simulink model "TST_Rail_MonMeUn"  (R2016b)
settings: Solver=FixedStepDiscrete  StartTime=0.0  StopTime=simTime  FixedStep=sampleTime  RelTol=1e-3
values from neighbouring files (symbols this model uses):
  testCase = 1    [initTST_Rail_MonMeUn_001.m]    (also in initTST_Rail_MonMeUn_002.m = 2; initTST_Rail_MonMeUn_003.m = 3; initTST_Rail_MonMeUn_004.m = 4; initTST_Rail_MonMeUn_005.m = 5)
libraries: simulink x91, UnitTest_Lib x81
(part 1 of 5)
settings Model: Creator=zhengjinyan  LastModifiedBy=zhengjinyan
settings DebuggingCC: SignalRangeChecking=error

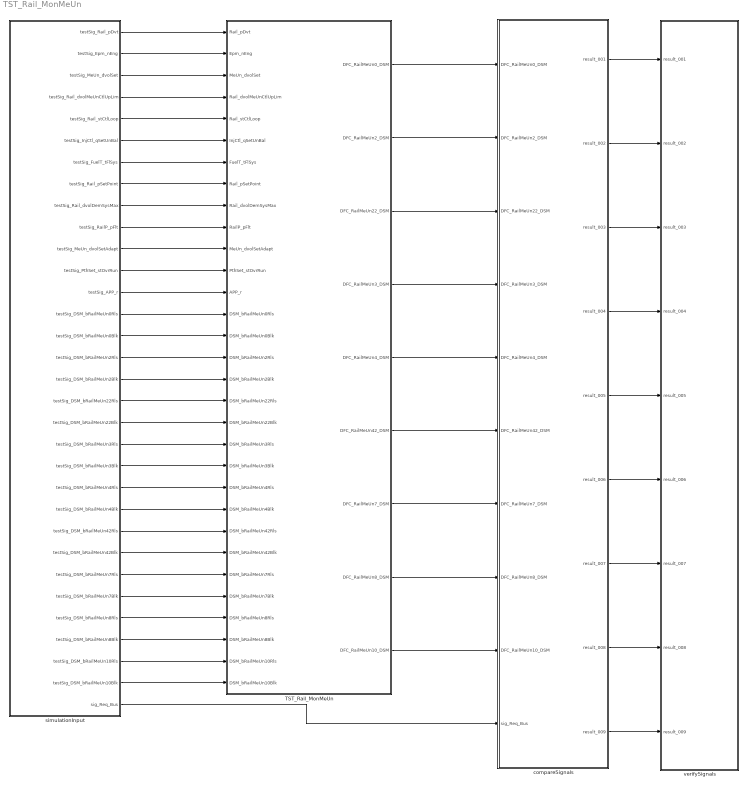
== system TST_Rail_MonMeUn ==
  TST_Rail_MonMeUn : Subsystem
  compareSignals : Subsystem
  simulationInput : Subsystem
  verifySignals : Subsystem
  wires:
  simulationInput/1(testSig_Rail_pDvt) -> TST_Rail_MonMeUn/1(Rail_pDvt)
  simulationInput/2(testSig_Epm_nEng) -> TST_Rail_MonMeUn/2(Epm_nEng)
  simulationInput/3(testSig_MeUn_dvolSet) -> TST_Rail_MonMeUn/3(MeUn_dvolSet)
  simulationInput/4(testSig_Rail_dvolMeUnCtlUpLim) -> TST_Rail_MonMeUn/4(Rail_dvolMeUnCtlUpLim)
  simulationInput/5(testSig_Rail_stCtlLoop) -> TST_Rail_MonMeUn/5(Rail_stCtlLoop)
  simulationInput/6(testSig_InjCtl_qSetUnBal) -> TST_Rail_MonMeUn/6(InjCtl_qSetUnBal)
  simulationInput/7(testSig_FuelT_tFlSys) -> TST_Rail_MonMeUn/7(FuelT_tFlSys)
  simulationInput/8(testSig_Rail_pSetPoint) -> TST_Rail_MonMeUn/8(Rail_pSetPoint)
  simulationInput/9(testSig_Rail_dvolDemSysMax) -> TST_Rail_MonMeUn/9(Rail_dvolDemSysMax)
  simulationInput/10(testSig_RailP_pFlt) -> TST_Rail_MonMeUn/10(RailP_pFlt)
  simulationInput/11(testSig_MeUn_dvolSetAdapt) -> TST_Rail_MonMeUn/11(MeUn_dvolSetAdapt)
  simulationInput/12(testSig_PthSet_stOvrRun) -> TST_Rail_MonMeUn/12(PthSet_stOvrRun)
  simulationInput/13(testSig_APP_r) -> TST_Rail_MonMeUn/13(APP_r)
  simulationInput/14(testSig_DSM_bRailMeUn0Rls) -> TST_Rail_MonMeUn/14(DSM_bRailMeUn0Rls)
  simulationInput/15(testSig_DSM_bRailMeUn0Blk) -> TST_Rail_MonMeUn/15(DSM_bRailMeUn0Blk)
  simulationInput/16(testSig_DSM_bRailMeUn2Rls) -> TST_Rail_MonMeUn/16(DSM_bRailMeUn2Rls)
  simulationInput/17(testSig_DSM_bRailMeUn2Blk) -> TST_Rail_MonMeUn/17(DSM_bRailMeUn2Blk)
  simulationInput/18(testSig_DSM_bRailMeUn22Rls) -> TST_Rail_MonMeUn/18(DSM_bRailMeUn22Rls)
  simulationInput/19(testSig_DSM_bRailMeUn22Blk) -> TST_Rail_MonMeUn/19(DSM_bRailMeUn22Blk)
  simulationInput/20(testSig_DSM_bRailMeUn3Rls) -> TST_Rail_MonMeUn/20(DSM_bRailMeUn3Rls)
  simulationInput/21(testSig_DSM_bRailMeUn3Blk) -> TST_Rail_MonMeUn/21(DSM_bRailMeUn3Blk)
  simulationInput/22(testSig_DSM_bRailMeUn4Rls) -> TST_Rail_MonMeUn/22(DSM_bRailMeUn4Rls)
  simulationInput/23(testSig_DSM_bRailMeUn4Blk) -> TST_Rail_MonMeUn/23(DSM_bRailMeUn4Blk)
  simulationInput/24(testSig_DSM_bRailMeUn42Rls) -> TST_Rail_MonMeUn/24(DSM_bRailMeUn42Rls)
  simulationInput/25(testSig_DSM_bRailMeUn42Blk) -> TST_Rail_MonMeUn/25(DSM_bRailMeUn42Blk)
  simulationInput/26(testSig_DSM_bRailMeUn7Rls) -> TST_Rail_MonMeUn/26(DSM_bRailMeUn7Rls)
  simulationInput/27(testSig_DSM_bRailMeUn7Blk) -> TST_Rail_MonMeUn/27(DSM_bRailMeUn7Blk)
  simulationInput/28(testSig_DSM_bRailMeUn8Rls) -> TST_Rail_MonMeUn/28(DSM_bRailMeUn8Rls)
  simulationInput/29(testSig_DSM_bRailMeUn8Blk) -> TST_Rail_MonMeUn/29(DSM_bRailMeUn8Blk)
  simulationInput/30(testSig_DSM_bRailMeUn10Rls) -> TST_Rail_MonMeUn/30(DSM_bRailMeUn10Rls)
  simulationInput/31(testSig_DSM_bRailMeUn10Blk) -> TST_Rail_MonMeUn/31(DSM_bRailMeUn10Blk)
  TST_Rail_MonMeUn/1(DFC_RailMeUn0_DSM) -> compareSignals/1(DFC_RailMeUn0_DSM)
  TST_Rail_MonMeUn/2(DFC_RailMeUn2_DSM) -> compareSignals/2(DFC_RailMeUn2_DSM)
  TST_Rail_MonMeUn/3(DFC_RailMeUn22_DSM) -> compareSignals/3(DFC_RailMeUn22_DSM)
  TST_Rail_MonMeUn/4(DFC_RailMeUn3_DSM) -> compareSignals/4(DFC_RailMeUn3_DSM)
  TST_Rail_MonMeUn/5(DFC_RailMeUn4_DSM) -> compareSignals/5(DFC_RailMeUn4_DSM)
  TST_Rail_MonMeUn/6(DFC_RailMeUn42_DSM) -> compareSignals/6(DFC_RailMeUn42_DSM)
  TST_Rail_MonMeUn/7(DFC_RailMeUn7_DSM) -> compareSignals/7(DFC_RailMeUn7_DSM)
  TST_Rail_MonMeUn/8(DFC_RailMeUn8_DSM) -> compareSignals/8(DFC_RailMeUn8_DSM)
  TST_Rail_MonMeUn/9(DFC_RailMeUn10_DSM) -> compareSignals/9(DFC_RailMeUn10_DSM)
  simulationInput/32(sig_Req_Bus) -> compareSignals/10(sig_Req_Bus)
  compareSignals/1(result_001) -> verifySignals/1(result_001)
  compareSignals/2(result_002) -> verifySignals/2(result_002)
  compareSignals/3(result_003) -> verifySignals/3(result_003)
  compareSignals/4(result_004) -> verifySignals/4(result_004)
  compareSignals/5(result_005) -> verifySignals/5(result_005)
  compareSignals/6(result_006) -> verifySignals/6(result_006)
  compareSignals/7(result_007) -> verifySignals/7(result_007)
  compareSignals/8(result_008) -> verifySignals/8(result_008)
  compareSignals/9(result_009) -> verifySignals/9(result_009)

== system TST_Rail_MonMeUn/TST_Rail_MonMeUn ==
  Rail_pDvt : Inport
  Epm_nEng : Inport  Port=2
  MeUn_dvolSet : Inport  Port=3
  Rail_dvolMeUnCtlUpLim : Inport  Port=4
  Rail_stCtlLoop : Inport  Port=5
  InjCtl_qSetUnBal : Inport  Port=6
  FuelT_tFlSys : Inport  Port=7
  Rail_pSetPoint : Inport  Port=8
  Rail_dvolDemSysMax : Inport  Port=9
  RailP_pFlt : Inport  Port=10
  MeUn_dvolSetAdapt : Inport  Port=11
  PthSet_stOvrRun : Inport  Port=12
  APP_r : Inport  Port=13
  DSM_bRailMeUn0Rls : Inport  Port=14
  DSM_bRailMeUn0Blk : Inport  Port=15
  DSM_bRailMeUn2Rls : Inport  Port=16
  DSM_bRailMeUn2Blk : Inport  Port=17
  DSM_bRailMeUn22Rls : Inport  Port=18
  DSM_bRailMeUn22Blk : Inport  Port=19
  DSM_bRailMeUn3Rls : Inport  Port=20
  DSM_bRailMeUn3Blk : Inport  Port=21
  DSM_bRailMeUn4Rls : Inport  Port=22
  DSM_bRailMeUn4Blk : Inport  Port=23
  DSM_bRailMeUn42Rls : Inport  Port=24
  DSM_bRailMeUn42Blk : Inport  Port=25
  DSM_bRailMeUn7Rls : Inport  Port=26
  DSM_bRailMeUn7Blk : Inport  Port=27
  DSM_bRailMeUn8Rls : Inport  Port=28
  DSM_bRailMeUn8Blk : Inport  Port=29
  DSM_bRailMeUn10Rls : Inport  Port=30
  DSM_bRailMeUn10Blk : Inport  Port=31
  Function_Call : simulink/Ports & Subsystems/Function-Call Generator  sample_time=sampleTime  numberOfIterations=1
  Rail_MonMeUn : ModelReference  ModelNameDialog=Rail_MonMeUn  SimulationMode=Normal  ModelReferenceVersion=1.32  TriggerPortName=function  TriggerPortTriggerType=function-call  TriggerPortStatesWhenEnabling=held
  DFC_RailMeUn0_DSM : Outport
  DFC_RailMeUn2_DSM : Outport  Port=2
  DFC_RailMeUn22_DSM : Outport  Port=3
  DFC_RailMeUn3_DSM : Outport  Port=4
  DFC_RailMeUn4_DSM : Outport  Port=5
  DFC_RailMeUn42_DSM : Outport  Port=6
  DFC_RailMeUn7_DSM : Outport  Port=7
  DFC_RailMeUn8_DSM : Outport  Port=8
  DFC_RailMeUn10_DSM : Outport  Port=9
  wires:
  Function_Call/1 -> Rail_MonMeUn/Trigger
  Rail_pDvt/1 -> Rail_MonMeUn/1
  Epm_nEng/1 -> Rail_MonMeUn/2
  MeUn_dvolSet/1 -> Rail_MonMeUn/3
  Rail_dvolMeUnCtlUpLim/1 -> Rail_MonMeUn/4
  Rail_stCtlLoop/1 -> Rail_MonMeUn/5
  InjCtl_qSetUnBal/1 -> Rail_MonMeUn/6
  FuelT_tFlSys/1 -> Rail_MonMeUn/7
  Rail_pSetPoint/1 -> Rail_MonMeUn/8
  Rail_dvolDemSysMax/1 -> Rail_MonMeUn/9
  RailP_pFlt/1 -> Rail_MonMeUn/10
  MeUn_dvolSetAdapt/1 -> Rail_MonMeUn/11
  PthSet_stOvrRun/1 -> Rail_MonMeUn/12
  APP_r/1 -> Rail_MonMeUn/13
  DSM_bRailMeUn0Rls/1 -> Rail_MonMeUn/14
  DSM_bRailMeUn0Blk/1 -> Rail_MonMeUn/15
  DSM_bRailMeUn2Rls/1 -> Rail_MonMeUn/16
  DSM_bRailMeUn2Blk/1 -> Rail_MonMeUn/17
  DSM_bRailMeUn22Rls/1 -> Rail_MonMeUn/18
  DSM_bRailMeUn22Blk/1 -> Rail_MonMeUn/19
  DSM_bRailMeUn3Rls/1 -> Rail_MonMeUn/20
  DSM_bRailMeUn3Blk/1 -> Rail_MonMeUn/21
  DSM_bRailMeUn4Rls/1 -> Rail_MonMeUn/22
  DSM_bRailMeUn4Blk/1 -> Rail_MonMeUn/23
  DSM_bRailMeUn42Rls/1 -> Rail_MonMeUn/24
  DSM_bRailMeUn42Blk/1 -> Rail_MonMeUn/25
  DSM_bRailMeUn7Rls/1 -> Rail_MonMeUn/26
  DSM_bRailMeUn7Blk/1 -> Rail_MonMeUn/27
  DSM_bRailMeUn8Rls/1 -> Rail_MonMeUn/28
  DSM_bRailMeUn8Blk/1 -> Rail_MonMeUn/29
  DSM_bRailMeUn10Rls/1 -> Rail_MonMeUn/30
  DSM_bRailMeUn10Blk/1 -> Rail_MonMeUn/31
  Rail_MonMeUn/1 -> DFC_RailMeUn0_DSM/1
  Rail_MonMeUn/2 -> DFC_RailMeUn2_DSM/1
  Rail_MonMeUn/3 -> DFC_RailMeUn22_DSM/1
  Rail_MonMeUn/4 -> DFC_RailMeUn3_DSM/1
  Rail_MonMeUn/5 -> DFC_RailMeUn4_DSM/1
  Rail_MonMeUn/6 -> DFC_RailMeUn42_DSM/1
  Rail_MonMeUn/7 -> DFC_RailMeUn7_DSM/1
  Rail_MonMeUn/8 -> DFC_RailMeUn8_DSM/1
  Rail_MonMeUn/9 -> DFC_RailMeUn10_DSM/1

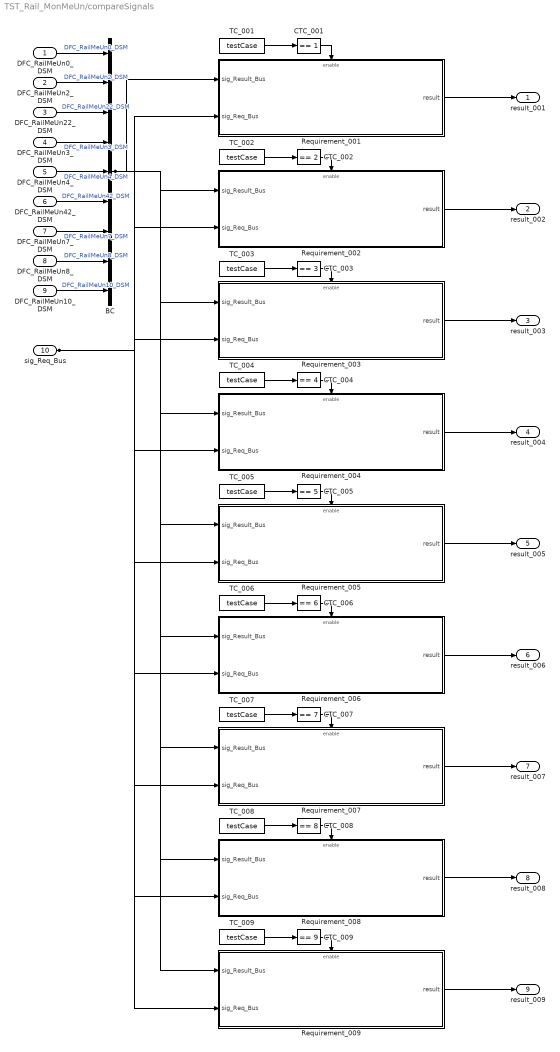
== system TST_Rail_MonMeUn/compareSignals ==
  DFC_RailMeUn0_DSM : Inport
  DFC_RailMeUn2_DSM : Inport  Port=2
  DFC_RailMeUn22_DSM : Inport  Port=3
  DFC_RailMeUn3_DSM : Inport  Port=4
  DFC_RailMeUn4_DSM : Inport  Port=5
  DFC_RailMeUn42_DSM : Inport  Port=6
  DFC_RailMeUn7_DSM : Inport  Port=7
  DFC_RailMeUn8_DSM : Inport  Port=8
  DFC_RailMeUn10_DSM : Inport  Port=9
  sig_Req_Bus : Inport  Port=10
  BC : BusCreator  Inputs=9
  CTC_001 : simulink/Logic and Bit Operations/Compare To Constant  relop===  const=1  OutDataTypeStr=boolean
  CTC_002 : simulink/Logic and Bit Operations/Compare To Constant  relop===  const=2  OutDataTypeStr=boolean
  CTC_003 : simulink/Logic and Bit Operations/Compare To Constant  relop===  const=3  OutDataTypeStr=boolean
  CTC_004 : simulink/Logic and Bit Operations/Compare To Constant  relop===  const=4  OutDataTypeStr=boolean
  CTC_005 : simulink/Logic and Bit Operations/Compare To Constant  relop===  const=5  OutDataTypeStr=boolean
  CTC_006 : simulink/Logic and Bit Operations/Compare To Constant  relop===  const=6  OutDataTypeStr=boolean
  CTC_007 : simulink/Logic and Bit Operations/Compare To Constant  relop===  const=7  OutDataTypeStr=boolean
  CTC_008 : simulink/Logic and Bit Operations/Compare To Constant  relop===  const=8  OutDataTypeStr=boolean
  CTC_009 : simulink/Logic and Bit Operations/Compare To Constant  relop===  const=9  OutDataTypeStr=boolean
  Requirement_001 : Subsystem
  Requirement_002 : Subsystem
  Requirement_003 : Subsystem
  Requirement_004 : Subsystem
  Requirement_005 : Subsystem
  Requirement_006 : Subsystem
  Requirement_007 : Subsystem
  Requirement_008 : Subsystem
  Requirement_009 : Subsystem
  TC_001 : Constant  Value=testCase
  TC_002 : Constant  Value=testCase
  TC_003 : Constant  Value=testCase
  TC_004 : Constant  Value=testCase
  TC_005 : Constant  Value=testCase
  TC_006 : Constant  Value=testCase
  TC_007 : Constant  Value=testCase
  TC_008 : Constant  Value=testCase
  TC_009 : Constant  Value=testCase
  result_001 : Outport
  result_002 : Outport  Port=2
  result_003 : Outport  Port=3
  result_004 : Outport  Port=4
  result_005 : Outport  Port=5
  result_006 : Outport  Port=6
  result_007 : Outport  Port=7
  result_008 : Outport  Port=8
  result_009 : Outport  Port=9
  wires:
  DFC_RailMeUn0_DSM/1 -> BC/1  "DFC_RailMeUn0_DSM"
  DFC_RailMeUn2_DSM/1 -> BC/2  "DFC_RailMeUn2_DSM"
  DFC_RailMeUn22_DSM/1 -> BC/3  "DFC_RailMeUn22_DSM"
  DFC_RailMeUn3_DSM/1 -> BC/4  "DFC_RailMeUn3_DSM"
  DFC_RailMeUn4_DSM/1 -> BC/5  "DFC_RailMeUn4_DSM"
  DFC_RailMeUn42_DSM/1 -> BC/6  "DFC_RailMeUn42_DSM"
  DFC_RailMeUn7_DSM/1 -> BC/7  "DFC_RailMeUn7_DSM"
  DFC_RailMeUn8_DSM/1 -> BC/8  "DFC_RailMeUn8_DSM"
  DFC_RailMeUn10_DSM/1 -> BC/9  "DFC_RailMeUn10_DSM"
  TC_001/1 -> CTC_001/1
  CTC_001/1 -> Requirement_001/Enable
  sig_Req_Bus/1 -> Requirement_001/2(sig_Req_Bus), Requirement_002/2(sig_Req_Bus), Requirement_003/2(sig_Req_Bus), Requirement_004/2(sig_Req_Bus), Requirement_005/2(sig_Req_Bus), Requirement_006/2(sig_Req_Bus), Requirement_007/2(sig_Req_Bus), Requirement_008/2(sig_Req_Bus), Requirement_009/2(sig_Req_Bus)
  BC/1 -> Requirement_001/1(sig_Result_Bus), Requirement_002/1(sig_Result_Bus), Requirement_003/1(sig_Result_Bus), Requirement_004/1(sig_Result_Bus), Requirement_005/1(sig_Result_Bus), Requirement_006/1(sig_Result_Bus), Requirement_007/1(sig_Result_Bus), Requirement_008/1(sig_Result_Bus), Requirement_009/1(sig_Result_Bus)
  Requirement_001/1(result) -> result_001/1
  TC_002/1 -> CTC_002/1
  CTC_002/1 -> Requirement_002/Enable
  Requirement_002/1(result) -> result_002/1
  TC_003/1 -> CTC_003/1
  CTC_003/1 -> Requirement_003/Enable
  Requirement_003/1(result) -> result_003/1
  TC_004/1 -> CTC_004/1
  CTC_004/1 -> Requirement_004/Enable
  Requirement_004/1(result) -> result_004/1
  TC_005/1 -> CTC_005/1
  CTC_005/1 -> Requirement_005/Enable
  Requirement_005/1(result) -> result_005/1
  TC_006/1 -> CTC_006/1
  CTC_006/1 -> Requirement_006/Enable
  Requirement_006/1(result) -> result_006/1
  TC_007/1 -> CTC_007/1
  CTC_007/1 -> Requirement_007/Enable
  Requirement_007/1(result) -> result_007/1
  TC_008/1 -> CTC_008/1
  CTC_008/1 -> Requirement_008/Enable
  Requirement_008/1(result) -> result_008/1
  TC_009/1 -> CTC_009/1
  CTC_009/1 -> Requirement_009/Enable
  Requirement_009/1(result) -> result_009/1

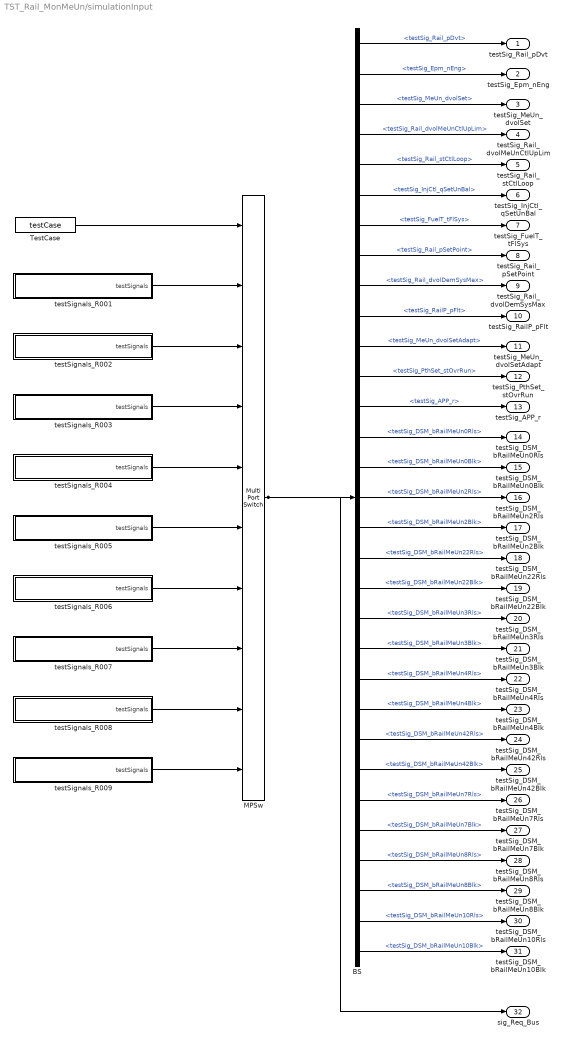
== system TST_Rail_MonMeUn/simulationInput ==
  BS : BusSelector  OutputSignals=testSig_Rail_pDvt,testSig_Epm_nEng,testSig_MeUn_dvolSet,testSig_Rail_dvolMeUnCtlUpLim,testSig_Rail_stCtlLoop,testSig_InjCtl_qSetUnBal,testSig_FuelT_tFlSys,testSig_Rail_pSetPoint,testSig_Rail_dvolDemSysMax,testSig_RailP_pFlt,testSig_MeUn_dvolSetAdapt,testSig_PthSet_stOvrRun,testSig_APP_r,testSig_DSM_bRailMeUn0Rls,testSig_DSM_bRailMeUn0Blk,testSig_DSM_bRailMeUn2Rls,testSig_DSM_bRailMeUn2Blk,testSig_DSM_bRailMeUn22Rls,testSig_DSM_bRailMeUn22Blk,testSig_DSM_bRailMeUn3Rls,testSig_DSM_bRailMeUn3Blk,testSig_DSM_bRailMeUn4Rls,testSig_DSM_bRailMeUn4Blk,testSig_DSM_bRailMeUn42Rls,testSig_DSM_bRailMeUn42Blk,testSig_DSM_bRailMeUn7Rls,testSig_DSM_bRailMeUn7Blk,testSig_DSM_bRailMeUn8Rls,testSig_DSM_bRailMeUn8Blk,testSig_DSM_bRailMeUn10Rls,testSig_DSM_bRailMeUn10Blk
  MPSw : MultiPortSwitch  Inputs=9  SaturateOnIntegerOverflow=on  InputSameDT=on
  TestCase : Constant  Value=testCase
  testSignals_R001 : Subsystem
  testSignals_R002 : Subsystem
  testSignals_R003 : Subsystem
  testSignals_R004 : Subsystem
  testSignals_R005 : Subsystem
  testSignals_R006 : Subsystem
  testSignals_R007 : Subsystem
  testSignals_R008 : Subsystem
  testSignals_R009 : Subsystem
  testSig_Rail_pDvt : Outport
  testSig_Epm_nEng : Outport  Port=2
  testSig_MeUn_dvolSet : Outport  Port=3
  testSig_Rail_dvolMeUnCtlUpLim : Outport  Port=4
  testSig_Rail_stCtlLoop : Outport  Port=5
  testSig_InjCtl_qSetUnBal : Outport  Port=6
  testSig_FuelT_tFlSys : Outport  Port=7
  testSig_Rail_pSetPoint : Outport  Port=8
  testSig_Rail_dvolDemSysMax : Outport  Port=9
  testSig_RailP_pFlt : Outport  Port=10
  testSig_MeUn_dvolSetAdapt : Outport  Port=11
  testSig_PthSet_stOvrRun : Outport  Port=12
  testSig_APP_r : Outport  Port=13
  testSig_DSM_bRailMeUn0Rls : Outport  Port=14
  testSig_DSM_bRailMeUn0Blk : Outport  Port=15
  testSig_DSM_bRailMeUn2Rls : Outport  Port=16
  testSig_DSM_bRailMeUn2Blk : Outport  Port=17
  testSig_DSM_bRailMeUn22Rls : Outport  Port=18
  testSig_DSM_bRailMeUn22Blk : Outport  Port=19
  testSig_DSM_bRailMeUn3Rls : Outport  Port=20
  testSig_DSM_bRailMeUn3Blk : Outport  Port=21
  testSig_DSM_bRailMeUn4Rls : Outport  Port=22
  testSig_DSM_bRailMeUn4Blk : Outport  Port=23
  testSig_DSM_bRailMeUn42Rls : Outport  Port=24
  testSig_DSM_bRailMeUn42Blk : Outport  Port=25
  testSig_DSM_bRailMeUn7Rls : Outport  Port=26
  testSig_DSM_bRailMeUn7Blk : Outport  Port=27
  testSig_DSM_bRailMeUn8Rls : Outport  Port=28
  testSig_DSM_bRailMeUn8Blk : Outport  Port=29
  testSig_DSM_bRailMeUn10Rls : Outport  Port=30
  testSig_DSM_bRailMeUn10Blk : Outport  Port=31
  sig_Req_Bus : Outport  Port=32
  wires:
  BS/1 -> testSig_Rail_pDvt/1  "<testSig_Rail_pDvt>"
  BS/2 -> testSig_Epm_nEng/1  "<testSig_Epm_nEng>"
  BS/3 -> testSig_MeUn_dvolSet/1  "<testSig_MeUn_dvolSet>"
  BS/4 -> testSig_Rail_dvolMeUnCtlUpLim/1  "<testSig_Rail_dvolMeUnCtlUpLim>"
  BS/5 -> testSig_Rail_stCtlLoop/1  "<testSig_Rail_stCtlLoop>"
  BS/6 -> testSig_InjCtl_qSetUnBal/1  "<testSig_InjCtl_qSetUnBal>"
  BS/7 -> testSig_FuelT_tFlSys/1  "<testSig_FuelT_tFlSys>"
  BS/8 -> testSig_Rail_pSetPoint/1  "<testSig_Rail_pSetPoint>"
  BS/9 -> testSig_Rail_dvolDemSysMax/1  "<testSig_Rail_dvolDemSysMax>"
  BS/10 -> testSig_RailP_pFlt/1  "<testSig_RailP_pFlt>"
  BS/11 -> testSig_MeUn_dvolSetAdapt/1  "<testSig_MeUn_dvolSetAdapt>"
  BS/12 -> testSig_PthSet_stOvrRun/1  "<testSig_PthSet_stOvrRun>"
  BS/13 -> testSig_APP_r/1  "<testSig_APP_r>"
  BS/14 -> testSig_DSM_bRailMeUn0Rls/1  "<testSig_DSM_bRailMeUn0Rls>"
  BS/15 -> testSig_DSM_bRailMeUn0Blk/1  "<testSig_DSM_bRailMeUn0Blk>"
  BS/16 -> testSig_DSM_bRailMeUn2Rls/1  "<testSig_DSM_bRailMeUn2Rls>"
  BS/17 -> testSig_DSM_bRailMeUn2Blk/1  "<testSig_DSM_bRailMeUn2Blk>"
  BS/18 -> testSig_DSM_bRailMeUn22Rls/1  "<testSig_DSM_bRailMeUn22Rls>"
  BS/19 -> testSig_DSM_bRailMeUn22Blk/1  "<testSig_DSM_bRailMeUn22Blk>"
  BS/20 -> testSig_DSM_bRailMeUn3Rls/1  "<testSig_DSM_bRailMeUn3Rls>"
  BS/21 -> testSig_DSM_bRailMeUn3Blk/1  "<testSig_DSM_bRailMeUn3Blk>"
  BS/22 -> testSig_DSM_bRailMeUn4Rls/1  "<testSig_DSM_bRailMeUn4Rls>"
  BS/23 -> testSig_DSM_bRailMeUn4Blk/1  "<testSig_DSM_bRailMeUn4Blk>"
  BS/24 -> testSig_DSM_bRailMeUn42Rls/1  "<testSig_DSM_bRailMeUn42Rls>"
  BS/25 -> testSig_DSM_bRailMeUn42Blk/1  "<testSig_DSM_bRailMeUn42Blk>"
  BS/26 -> testSig_DSM_bRailMeUn7Rls/1  "<testSig_DSM_bRailMeUn7Rls>"
  BS/27 -> testSig_DSM_bRailMeUn7Blk/1  "<testSig_DSM_bRailMeUn7Blk>"
  BS/28 -> testSig_DSM_bRailMeUn8Rls/1  "<testSig_DSM_bRailMeUn8Rls>"
  BS/29 -> testSig_DSM_bRailMeUn8Blk/1  "<testSig_DSM_bRailMeUn8Blk>"
  BS/30 -> testSig_DSM_bRailMeUn10Rls/1  "<testSig_DSM_bRailMeUn10Rls>"
  BS/31 -> testSig_DSM_bRailMeUn10Blk/1  "<testSig_DSM_bRailMeUn10Blk>"
  MPSw/1 -> BS/1, sig_Req_Bus/1
  TestCase/1 -> MPSw/1
  testSignals_R001/1(testSignals) -> MPSw/2
  testSignals_R002/1(testSignals) -> MPSw/3
  testSignals_R003/1(testSignals) -> MPSw/4
  testSignals_R004/1(testSignals) -> MPSw/5
  testSignals_R005/1(testSignals) -> MPSw/6
  testSignals_R006/1(testSignals) -> MPSw/7
  testSignals_R007/1(testSignals) -> MPSw/8
  testSignals_R008/1(testSignals) -> MPSw/9
  testSignals_R009/1(testSignals) -> MPSw/10

== system TST_Rail_MonMeUn/verifySignals ==
  result_001 : Inport
  result_002 : Inport  Port=2
  result_003 : Inport  Port=3
  result_004 : Inport  Port=4
  result_005 : Inport  Port=5
  result_006 : Inport  Port=6
  result_007 : Inport  Port=7
  result_008 : Inport  Port=8
  result_009 : Inport  Port=9
  Assertion_001 : Assertion  Enabled=off
  Assertion_002 : Assertion  Enabled=off
  Assertion_003 : Assertion  Enabled=off
  Assertion_004 : Assertion  Enabled=off
  Assertion_005 : Assertion  Enabled=off
  Assertion_006 : Assertion  Enabled=off
  Assertion_007 : Assertion  Enabled=off
  Assertion_008 : Assertion  Enabled=off
  Assertion_009 : Assertion  Enabled=off
  wires:
  result_001/1 -> Assertion_001/1
  result_002/1 -> Assertion_002/1
  result_003/1 -> Assertion_003/1
  result_004/1 -> Assertion_004/1
  result_005/1 -> Assertion_005/1
  result_006/1 -> Assertion_006/1
  result_007/1 -> Assertion_007/1
  result_008/1 -> Assertion_008/1
  result_009/1 -> Assertion_009/1

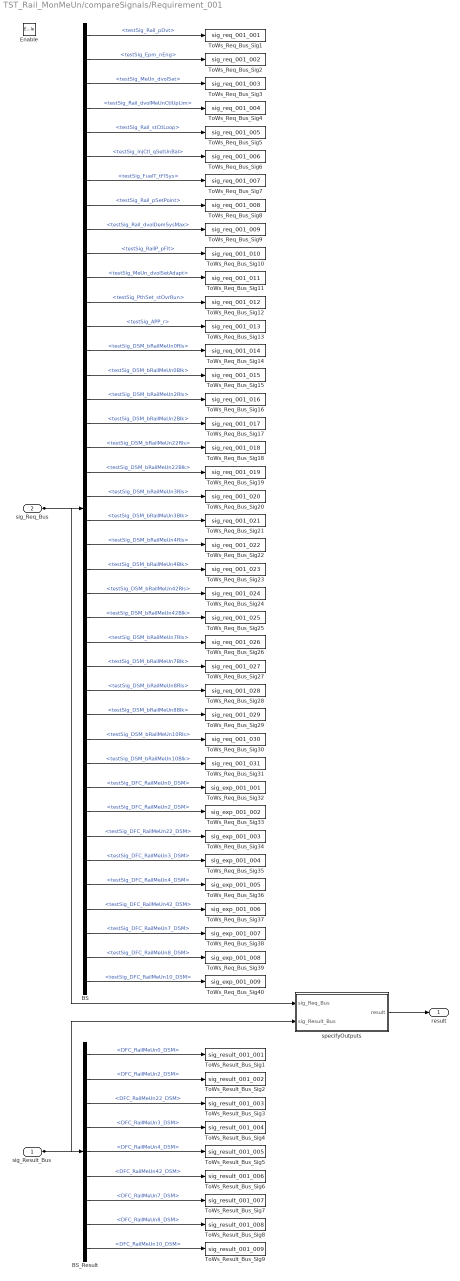
== system TST_Rail_MonMeUn/compareSignals/Requirement_001 ==
  sig_Result_Bus : Inport
  sig_Req_Bus : Inport  Port=2
  Enable : EnablePort
  BS : BusSelector  OutputSignals=testSig_Rail_pDvt,testSig_Epm_nEng,testSig_MeUn_dvolSet,testSig_Rail_dvolMeUnCtlUpLim,testSig_Rail_stCtlLoop,testSig_InjCtl_qSetUnBal,testSig_FuelT_tFlSys,testSig_Rail_pSetPoint,testSig_Rail_dvolDemSysMax,testSig_RailP_pFlt,testSig_MeUn_dvolSetAdapt,testSig_PthSet_stOvrRun,testSig_APP_r,testSig_DSM_bRailMeUn0Rls,testSig_DSM_bRailMeUn0Blk,testSig_DSM_bRailMeUn2Rls,testSig_DSM_bRailMeUn2Blk,testSig_DSM_bRailMeUn22Rls,testSig_DSM_bRailMeUn22Blk,testSig_DSM_bRailMeUn3Rls,testSig_DSM_bRailMeUn3Blk,testSig_DSM_bRailMeUn4Rls,testSig_DSM_bRailMeUn4Blk,testSig_DSM_bRailMeUn42Rls,testSig_DSM_bRailMeUn42Blk,testSig_DSM_bRailMeUn7Rls,testSig_DSM_bRailMeUn7Blk,testSig_DSM_bRailMeUn8Rls,testSig_DSM_bRailMeUn8Blk,testSig_DSM_bRailMeUn10Rls,testSig_DSM_bRailMeUn10Blk,testSig_DFC_RailMeUn0_DSM,testSig_DFC_RailMeUn2_DSM,testSig_DFC_RailMeUn22_DSM,testSig_DFC_RailMeUn3_DSM,testSig_DFC_RailMeUn4_DSM,testSig_DFC_RailMeUn42_DSM,testSig_DFC_RailMeUn7_DSM,testSig_DFC_RailMeUn8_DSM,testSig_DFC_RailMeUn10_DSM
  BS_Result : BusSelector  OutputSignals=DFC_RailMeUn0_DSM,DFC_RailMeUn2_DSM,DFC_RailMeUn22_DSM,DFC_RailMeUn3_DSM,DFC_RailMeUn4_DSM,DFC_RailMeUn42_DSM,DFC_RailMeUn7_DSM,DFC_RailMeUn8_DSM,DFC_RailMeUn10_DSM
  ToWs_Req_Bus_Sig1 : ToWorkspace  VariableName=sig_req_001_001  SaveFormat=Structure With Time
  ToWs_Req_Bus_Sig10 : ToWorkspace  VariableName=sig_req_001_010  SaveFormat=Structure With Time
  ToWs_Req_Bus_Sig11 : ToWorkspace  VariableName=sig_req_001_011  SaveFormat=Structure With Time
  ToWs_Req_Bus_Sig12 : ToWorkspace  VariableName=sig_req_001_012  SaveFormat=Structure With Time
  ToWs_Req_Bus_Sig13 : ToWorkspace  VariableName=sig_req_001_013  SaveFormat=Structure With Time
  ToWs_Req_Bus_Sig14 : ToWorkspace  VariableName=sig_req_001_014  SaveFormat=Structure With Time
  ToWs_Req_Bus_Sig15 : ToWorkspace  VariableName=sig_req_001_015  SaveFormat=Structure With Time
  ToWs_Req_Bus_Sig16 : ToWorkspace  VariableName=sig_req_001_016  SaveFormat=Structure With Time
  ToWs_Req_Bus_Sig17 : ToWorkspace  VariableName=sig_req_001_017  SaveFormat=Structure With Time
  ToWs_Req_Bus_Sig18 : ToWorkspace  VariableName=sig_req_001_018  SaveFormat=Structure With Time
  ToWs_Req_Bus_Sig19 : ToWorkspace  VariableName=sig_req_001_019  SaveFormat=Structure With Time
  ToWs_Req_Bus_Sig2 : ToWorkspace  VariableName=sig_req_001_002  SaveFormat=Structure With Time
  ToWs_Req_Bus_Sig20 : ToWorkspace  VariableName=sig_req_001_020  SaveFormat=Structure With Time
  ToWs_Req_Bus_Sig21 : ToWorkspace  VariableName=sig_req_001_021  SaveFormat=Structure With Time
  ToWs_Req_Bus_Sig22 : ToWorkspace  VariableName=sig_req_001_022  SaveFormat=Structure With Time
  ToWs_Req_Bus_Sig23 : ToWorkspace  VariableName=sig_req_001_023  SaveFormat=Structure With Time
  ToWs_Req_Bus_Sig24 : ToWorkspace  VariableName=sig_req_001_024  SaveFormat=Structure With Time
  ToWs_Req_Bus_Sig25 : ToWorkspace  VariableName=sig_req_001_025  SaveFormat=Structure With Time
  ToWs_Req_Bus_Sig26 : ToWorkspace  VariableName=sig_req_001_026  SaveFormat=Structure With Time
  ToWs_Req_Bus_Sig27 : ToWorkspace  VariableName=sig_req_001_027  SaveFormat=Structure With Time
  ToWs_Req_Bus_Sig28 : ToWorkspace  VariableName=sig_req_001_028  SaveFormat=Structure With Time
  ToWs_Req_Bus_Sig29 : ToWorkspace  VariableName=sig_req_001_029  SaveFormat=Structure With Time
  ToWs_Req_Bus_Sig3 : ToWorkspace  VariableName=sig_req_001_003  SaveFormat=Structure With Time
  ToWs_Req_Bus_Sig30 : ToWorkspace  VariableName=sig_req_001_030  SaveFormat=Structure With Time
  ToWs_Req_Bus_Sig31 : ToWorkspace  VariableName=sig_req_001_031  SaveFormat=Structure With Time
  ToWs_Req_Bus_Sig32 : ToWorkspace  VariableName=sig_exp_001_001  SaveFormat=Structure With Time
  ToWs_Req_Bus_Sig33 : ToWorkspace  VariableName=sig_exp_001_002  SaveFormat=Structure With Time
  ToWs_Req_Bus_Sig34 : ToWorkspace  VariableName=sig_exp_001_003  SaveFormat=Structure With Time
  ToWs_Req_Bus_Sig35 : ToWorkspace  VariableName=sig_exp_001_004  SaveFormat=Structure With Time
  ToWs_Req_Bus_Sig36 : ToWorkspace  VariableName=sig_exp_001_005  SaveFormat=Structure With Time
  ToWs_Req_Bus_Sig37 : ToWorkspace  VariableName=sig_exp_001_006  SaveFormat=Structure With Time
  ToWs_Req_Bus_Sig38 : ToWorkspace  VariableName=sig_exp_001_007  SaveFormat=Structure With Time
  ToWs_Req_Bus_Sig39 : ToWorkspace  VariableName=sig_exp_001_008  SaveFormat=Structure With Time
  ToWs_Req_Bus_Sig4 : ToWorkspace  VariableName=sig_req_001_004  SaveFormat=Structure With Time
  ToWs_Req_Bus_Sig40 : ToWorkspace  VariableName=sig_exp_001_009  SaveFormat=Structure With Time
  ToWs_Req_Bus_Sig5 : ToWorkspace  VariableName=sig_req_001_005  SaveFormat=Structure With Time
  ToWs_Req_Bus_Sig6 : ToWorkspace  VariableName=sig_req_001_006  SaveFormat=Structure With Time
  ToWs_Req_Bus_Sig7 : ToWorkspace  VariableName=sig_req_001_007  SaveFormat=Structure With Time
  ToWs_Req_Bus_Sig8 : ToWorkspace  VariableName=sig_req_001_008  SaveFormat=Structure With Time
  ToWs_Req_Bus_Sig9 : ToWorkspace  VariableName=sig_req_001_009  SaveFormat=Structure With Time
  ToWs_Result_Bus_Sig1 : ToWorkspace  VariableName=sig_result_001_001  SaveFormat=Structure With Time
  ToWs_Result_Bus_Sig2 : ToWorkspace  VariableName=sig_result_001_002  SaveFormat=Structure With Time
  ToWs_Result_Bus_Sig3 : ToWorkspace  VariableName=sig_result_001_003  SaveFormat=Structure With Time
  ToWs_Result_Bus_Sig4 : ToWorkspace  VariableName=sig_result_001_004  SaveFormat=Structure With Time
  ToWs_Result_Bus_Sig5 : ToWorkspace  VariableName=sig_result_001_005  SaveFormat=Structure With Time
  ToWs_Result_Bus_Sig6 : ToWorkspace  VariableName=sig_result_001_006  SaveFormat=Structure With Time
  ToWs_Result_Bus_Sig7 : ToWorkspace  VariableName=sig_result_001_007  SaveFormat=Structure With Time
  ToWs_Result_Bus_Sig8 : ToWorkspace  VariableName=sig_result_001_008  SaveFormat=Structure With Time
  ToWs_Result_Bus_Sig9 : ToWorkspace  VariableName=sig_result_001_009  SaveFormat=Structure With Time
  specifyOutputs : Subsystem
  result : Outport
  wires:
  sig_Req_Bus/1 -> BS/1, specifyOutputs/1(sig_Req_Bus)
  BS/1 -> ToWs_Req_Bus_Sig1/1  "<testSig_Rail_pDvt>"
  BS/2 -> ToWs_Req_Bus_Sig2/1  "<testSig_Epm_nEng>"
  BS/3 -> ToWs_Req_Bus_Sig3/1  "<testSig_MeUn_dvolSet>"
  BS/4 -> ToWs_Req_Bus_Sig4/1  "<testSig_Rail_dvolMeUnCtlUpLim>"
  BS/5 -> ToWs_Req_Bus_Sig5/1  "<testSig_Rail_stCtlLoop>"
  BS/6 -> ToWs_Req_Bus_Sig6/1  "<testSig_InjCtl_qSetUnBal>"
  BS/7 -> ToWs_Req_Bus_Sig7/1  "<testSig_FuelT_tFlSys>"
  BS/8 -> ToWs_Req_Bus_Sig8/1  "<testSig_Rail_pSetPoint>"
  BS/9 -> ToWs_Req_Bus_Sig9/1  "<testSig_Rail_dvolDemSysMax>"
  BS/10 -> ToWs_Req_Bus_Sig10/1  "<testSig_RailP_pFlt>"
  BS/11 -> ToWs_Req_Bus_Sig11/1  "<testSig_MeUn_dvolSetAdapt>"
  BS/12 -> ToWs_Req_Bus_Sig12/1  "<testSig_PthSet_stOvrRun>"
  BS/13 -> ToWs_Req_Bus_Sig13/1  "<testSig_APP_r>"
  BS/14 -> ToWs_Req_Bus_Sig14/1  "<testSig_DSM_bRailMeUn0Rls>"
  BS/15 -> ToWs_Req_Bus_Sig15/1  "<testSig_DSM_bRailMeUn0Blk>"
  BS/16 -> ToWs_Req_Bus_Sig16/1  "<testSig_DSM_bRailMeUn2Rls>"
  BS/17 -> ToWs_Req_Bus_Sig17/1  "<testSig_DSM_bRailMeUn2Blk>"
  BS/18 -> ToWs_Req_Bus_Sig18/1  "<testSig_DSM_bRailMeUn22Rls>"
  BS/19 -> ToWs_Req_Bus_Sig19/1  "<testSig_DSM_bRailMeUn22Blk>"
  BS/20 -> ToWs_Req_Bus_Sig20/1  "<testSig_DSM_bRailMeUn3Rls>"
  BS/21 -> ToWs_Req_Bus_Sig21/1  "<testSig_DSM_bRailMeUn3Blk>"
  BS/22 -> ToWs_Req_Bus_Sig22/1  "<testSig_DSM_bRailMeUn4Rls>"
  BS/23 -> ToWs_Req_Bus_Sig23/1  "<testSig_DSM_bRailMeUn4Blk>"
  BS/24 -> ToWs_Req_Bus_Sig24/1  "<testSig_DSM_bRailMeUn42Rls>"
  BS/25 -> ToWs_Req_Bus_Sig25/1  "<testSig_DSM_bRailMeUn42Blk>"
  BS/26 -> ToWs_Req_Bus_Sig26/1  "<testSig_DSM_bRailMeUn7Rls>"
  BS/27 -> ToWs_Req_Bus_Sig27/1  "<testSig_DSM_bRailMeUn7Blk>"
  BS/28 -> ToWs_Req_Bus_Sig28/1  "<testSig_DSM_bRailMeUn8Rls>"
  BS/29 -> ToWs_Req_Bus_Sig29/1  "<testSig_DSM_bRailMeUn8Blk>"
  BS/30 -> ToWs_Req_Bus_Sig30/1  "<testSig_DSM_bRailMeUn10Rls>"
  BS/31 -> ToWs_Req_Bus_Sig31/1  "<testSig_DSM_bRailMeUn10Blk>"
  BS/32 -> ToWs_Req_Bus_Sig32/1  "<testSig_DFC_RailMeUn0_DSM>"
  BS/33 -> ToWs_Req_Bus_Sig33/1  "<testSig_DFC_RailMeUn2_DSM>"
  BS/34 -> ToWs_Req_Bus_Sig34/1  "<testSig_DFC_RailMeUn22_DSM>"
  BS/35 -> ToWs_Req_Bus_Sig35/1  "<testSig_DFC_RailMeUn3_DSM>"
  BS/36 -> ToWs_Req_Bus_Sig36/1  "<testSig_DFC_RailMeUn4_DSM>"
  BS/37 -> ToWs_Req_Bus_Sig37/1  "<testSig_DFC_RailMeUn42_DSM>"
  BS/38 -> ToWs_Req_Bus_Sig38/1  "<testSig_DFC_RailMeUn7_DSM>"
  BS/39 -> ToWs_Req_Bus_Sig39/1  "<testSig_DFC_RailMeUn8_DSM>"
  BS/40 -> ToWs_Req_Bus_Sig40/1  "<testSig_DFC_RailMeUn10_DSM>"
  sig_Result_Bus/1 -> BS_Result/1, specifyOutputs/2(sig_Result_Bus)
  BS_Result/1 -> ToWs_Result_Bus_Sig1/1  "<DFC_RailMeUn0_DSM>"
  BS_Result/2 -> ToWs_Result_Bus_Sig2/1  "<DFC_RailMeUn2_DSM>"
  BS_Result/3 -> ToWs_Result_Bus_Sig3/1  "<DFC_RailMeUn22_DSM>"
  BS_Result/4 -> ToWs_Result_Bus_Sig4/1  "<DFC_RailMeUn3_DSM>"
  BS_Result/5 -> ToWs_Result_Bus_Sig5/1  "<DFC_RailMeUn4_DSM>"
  BS_Result/6 -> ToWs_Result_Bus_Sig6/1  "<DFC_RailMeUn42_DSM>"
  BS_Result/7 -> ToWs_Result_Bus_Sig7/1  "<DFC_RailMeUn7_DSM>"
  BS_Result/8 -> ToWs_Result_Bus_Sig8/1  "<DFC_RailMeUn8_DSM>"
  BS_Result/9 -> ToWs_Result_Bus_Sig9/1  "<DFC_RailMeUn10_DSM>"
  specifyOutputs/1(result) -> result/1

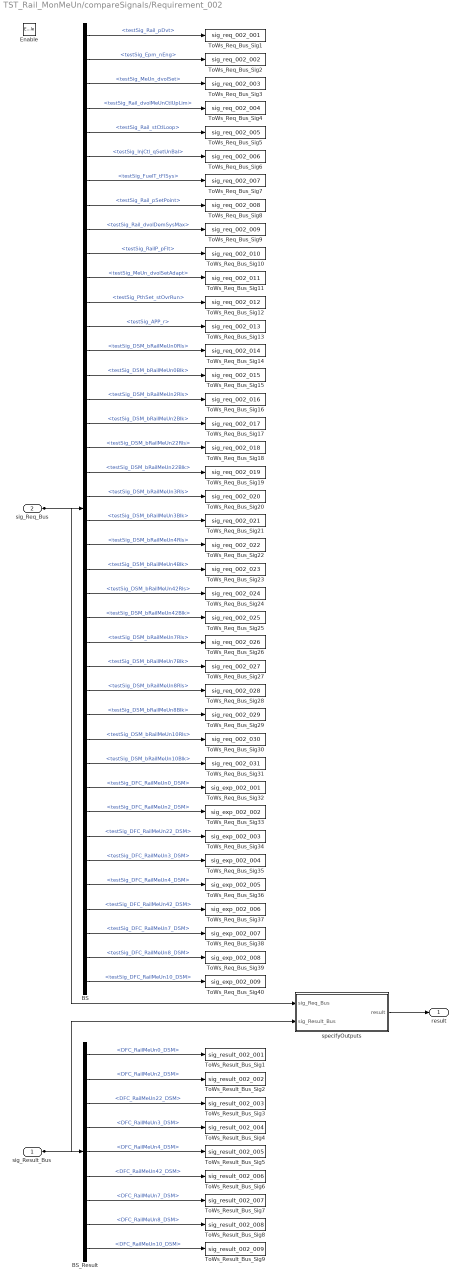
== system TST_Rail_MonMeUn/compareSignals/Requirement_002 ==
  sig_Result_Bus : Inport
  sig_Req_Bus : Inport  Port=2
  Enable : EnablePort
  BS : BusSelector  OutputSignals=testSig_Rail_pDvt,testSig_Epm_nEng,testSig_MeUn_dvolSet,testSig_Rail_dvolMeUnCtlUpLim,testSig_Rail_stCtlLoop,testSig_InjCtl_qSetUnBal,testSig_FuelT_tFlSys,testSig_Rail_pSetPoint,testSig_Rail_dvolDemSysMax,testSig_RailP_pFlt,testSig_MeUn_dvolSetAdapt,testSig_PthSet_stOvrRun,testSig_APP_r,testSig_DSM_bRailMeUn0Rls,testSig_DSM_bRailMeUn0Blk,testSig_DSM_bRailMeUn2Rls,testSig_DSM_bRailMeUn2Blk,testSig_DSM_bRailMeUn22Rls,testSig_DSM_bRailMeUn22Blk,testSig_DSM_bRailMeUn3Rls,testSig_DSM_bRailMeUn3Blk,testSig_DSM_bRailMeUn4Rls,testSig_DSM_bRailMeUn4Blk,testSig_DSM_bRailMeUn42Rls,testSig_DSM_bRailMeUn42Blk,testSig_DSM_bRailMeUn7Rls,testSig_DSM_bRailMeUn7Blk,testSig_DSM_bRailMeUn8Rls,testSig_DSM_bRailMeUn8Blk,testSig_DSM_bRailMeUn10Rls,testSig_DSM_bRailMeUn10Blk,testSig_DFC_RailMeUn0_DSM,testSig_DFC_RailMeUn2_DSM,testSig_DFC_RailMeUn22_DSM,testSig_DFC_RailMeUn3_DSM,testSig_DFC_RailMeUn4_DSM,testSig_DFC_RailMeUn42_DSM,testSig_DFC_RailMeUn7_DSM,testSig_DFC_RailMeUn8_DSM,testSig_DFC_RailMeUn10_DSM
  BS_Result : BusSelector  OutputSignals=DFC_RailMeUn0_DSM,DFC_RailMeUn2_DSM,DFC_RailMeUn22_DSM,DFC_RailMeUn3_DSM,DFC_RailMeUn4_DSM,DFC_RailMeUn42_DSM,DFC_RailMeUn7_DSM,DFC_RailMeUn8_DSM,DFC_RailMeUn10_DSM
  ToWs_Req_Bus_Sig1 : ToWorkspace  VariableName=sig_req_002_001  SaveFormat=Structure With Time
  ToWs_Req_Bus_Sig10 : ToWorkspace  VariableName=sig_req_002_010  SaveFormat=Structure With Time
  ToWs_Req_Bus_Sig11 : ToWorkspace  VariableName=sig_req_002_011  SaveFormat=Structure With Time
  ToWs_Req_Bus_Sig12 : ToWorkspace  VariableName=sig_req_002_012  SaveFormat=Structure With Time
  ToWs_Req_Bus_Sig13 : ToWorkspace  VariableName=sig_req_002_013  SaveFormat=Structure With Time
  ToWs_Req_Bus_Sig14 : ToWorkspace  VariableName=sig_req_002_014  SaveFormat=Structure With Time
  ToWs_Req_Bus_Sig15 : ToWorkspace  VariableName=sig_req_002_015  SaveFormat=Structure With Time
  ToWs_Req_Bus_Sig16 : ToWorkspace  VariableName=sig_req_002_016  SaveFormat=Structure With Time
  ToWs_Req_Bus_Sig17 : ToWorkspace  VariableName=sig_req_002_017  SaveFormat=Structure With Time
  ToWs_Req_Bus_Sig18 : ToWorkspace  VariableName=sig_req_002_018  SaveFormat=Structure With Time
  ToWs_Req_Bus_Sig19 : ToWorkspace  VariableName=sig_req_002_019  SaveFormat=Structure With Time
  ToWs_Req_Bus_Sig2 : ToWorkspace  VariableName=sig_req_002_002  SaveFormat=Structure With Time
  ToWs_Req_Bus_Sig20 : ToWorkspace  VariableName=sig_req_002_020  SaveFormat=Structure With Time
  ToWs_Req_Bus_Sig21 : ToWorkspace  VariableName=sig_req_002_021  SaveFormat=Structure With Time
  ToWs_Req_Bus_Sig22 : ToWorkspace  VariableName=sig_req_002_022  SaveFormat=Structure With Time
  ToWs_Req_Bus_Sig23 : ToWorkspace  VariableName=sig_req_002_023  SaveFormat=Structure With Time
  ToWs_Req_Bus_Sig24 : ToWorkspace  VariableName=sig_req_002_024  SaveFormat=Structure With Time
  ToWs_Req_Bus_Sig25 : ToWorkspace  VariableName=sig_req_002_025  SaveFormat=Structure With Time
  ToWs_Req_Bus_Sig26 : ToWorkspace  VariableName=sig_req_002_026  SaveFormat=Structure With Time
  ToWs_Req_Bus_Sig27 : ToWorkspace  VariableName=sig_req_002_027  SaveFormat=Structure With Time
  ToWs_Req_Bus_Sig28 : ToWorkspace  VariableName=sig_req_002_028  SaveFormat=Structure With Time
  ToWs_Req_Bus_Sig29 : ToWorkspace  VariableName=sig_req_002_029  SaveFormat=Structure With Time
  ToWs_Req_Bus_Sig3 : ToWorkspace  VariableName=sig_req_002_003  SaveFormat=Structure With Time
  ToWs_Req_Bus_Sig30 : ToWorkspace  VariableName=sig_req_002_030  SaveFormat=Structure With Time
  ToWs_Req_Bus_Sig31 : ToWorkspace  VariableName=sig_req_002_031  SaveFormat=Structure With Time
  ToWs_Req_Bus_Sig32 : ToWorkspace  VariableName=sig_exp_002_001  SaveFormat=Structure With Time
  ToWs_Req_Bus_Sig33 : ToWorkspace  VariableName=sig_exp_002_002  SaveFormat=Structure With Time
  ToWs_Req_Bus_Sig34 : ToWorkspace  VariableName=sig_exp_002_003  SaveFormat=Structure With Time
  ToWs_Req_Bus_Sig35 : ToWorkspace  VariableName=sig_exp_002_004  SaveFormat=Structure With Time
  ToWs_Req_Bus_Sig36 : ToWorkspace  VariableName=sig_exp_002_005  SaveFormat=Structure With Time
  ToWs_Req_Bus_Sig37 : ToWorkspace  VariableName=sig_exp_002_006  SaveFormat=Structure With Time
  ToWs_Req_Bus_Sig38 : ToWorkspace  VariableName=sig_exp_002_007  SaveFormat=Structure With Time
  ToWs_Req_Bus_Sig39 : ToWorkspace  VariableName=sig_exp_002_008  SaveFormat=Structure With Time
  ToWs_Req_Bus_Sig4 : ToWorkspace  VariableName=sig_req_002_004  SaveFormat=Structure With Time
  ToWs_Req_Bus_Sig40 : ToWorkspace  VariableName=sig_exp_002_009  SaveFormat=Structure With Time
  ToWs_Req_Bus_Sig5 : ToWorkspace  VariableName=sig_req_002_005  SaveFormat=Structure With Time
  ToWs_Req_Bus_Sig6 : ToWorkspace  VariableName=sig_req_002_006  SaveFormat=Structure With Time
  ToWs_Req_Bus_Sig7 : ToWorkspace  VariableName=sig_req_002_007  SaveFormat=Structure With Time
  ToWs_Req_Bus_Sig8 : ToWorkspace  VariableName=sig_req_002_008  SaveFormat=Structure With Time
  ToWs_Req_Bus_Sig9 : ToWorkspace  VariableName=sig_req_002_009  SaveFormat=Structure With Time
  ToWs_Result_Bus_Sig1 : ToWorkspace  VariableName=sig_result_002_001  SaveFormat=Structure With Time
  ToWs_Result_Bus_Sig2 : ToWorkspace  VariableName=sig_result_002_002  SaveFormat=Structure With Time
  ToWs_Result_Bus_Sig3 : ToWorkspace  VariableName=sig_result_002_003  SaveFormat=Structure With Time
  ToWs_Result_Bus_Sig4 : ToWorkspace  VariableName=sig_result_002_004  SaveFormat=Structure With Time
  ToWs_Result_Bus_Sig5 : ToWorkspace  VariableName=sig_result_002_005  SaveFormat=Structure With Time
  ToWs_Result_Bus_Sig6 : ToWorkspace  VariableName=sig_result_002_006  SaveFormat=Structure With Time
  ToWs_Result_Bus_Sig7 : ToWorkspace  VariableName=sig_result_002_007  SaveFormat=Structure With Time
  ToWs_Result_Bus_Sig8 : ToWorkspace  VariableName=sig_result_002_008  SaveFormat=Structure With Time
  ToWs_Result_Bus_Sig9 : ToWorkspace  VariableName=sig_result_002_009  SaveFormat=Structure With Time
  specifyOutputs : Subsystem
  result : Outport
  wires:
  sig_Req_Bus/1 -> BS/1, specifyOutputs/1(sig_Req_Bus)
  BS/1 -> ToWs_Req_Bus_Sig1/1  "<testSig_Rail_pDvt>"
  BS/2 -> ToWs_Req_Bus_Sig2/1  "<testSig_Epm_nEng>"
  BS/3 -> ToWs_Req_Bus_Sig3/1  "<testSig_MeUn_dvolSet>"
  BS/4 -> ToWs_Req_Bus_Sig4/1  "<testSig_Rail_dvolMeUnCtlUpLim>"
  BS/5 -> ToWs_Req_Bus_Sig5/1  "<testSig_Rail_stCtlLoop>"
  BS/6 -> ToWs_Req_Bus_Sig6/1  "<testSig_InjCtl_qSetUnBal>"
  BS/7 -> ToWs_Req_Bus_Sig7/1  "<testSig_FuelT_tFlSys>"
  BS/8 -> ToWs_Req_Bus_Sig8/1  "<testSig_Rail_pSetPoint>"
  BS/9 -> ToWs_Req_Bus_Sig9/1  "<testSig_Rail_dvolDemSysMax>"
  BS/10 -> ToWs_Req_Bus_Sig10/1  "<testSig_RailP_pFlt>"
  BS/11 -> ToWs_Req_Bus_Sig11/1  "<testSig_MeUn_dvolSetAdapt>"
  BS/12 -> ToWs_Req_Bus_Sig12/1  "<testSig_PthSet_stOvrRun>"
  BS/13 -> ToWs_Req_Bus_Sig13/1  "<testSig_APP_r>"
  BS/14 -> ToWs_Req_Bus_Sig14/1  "<testSig_DSM_bRailMeUn0Rls>"
  BS/15 -> ToWs_Req_Bus_Sig15/1  "<testSig_DSM_bRailMeUn0Blk>"
  BS/16 -> ToWs_Req_Bus_Sig16/1  "<testSig_DSM_bRailMeUn2Rls>"
  BS/17 -> ToWs_Req_Bus_Sig17/1  "<testSig_DSM_bRailMeUn2Blk>"
  BS/18 -> ToWs_Req_Bus_Sig18/1  "<testSig_DSM_bRailMeUn22Rls>"
  BS/19 -> ToWs_Req_Bus_Sig19/1  "<testSig_DSM_bRailMeUn22Blk>"
  BS/20 -> ToWs_Req_Bus_Sig20/1  "<testSig_DSM_bRailMeUn3Rls>"
  BS/21 -> ToWs_Req_Bus_Sig21/1  "<testSig_DSM_bRailMeUn3Blk>"
  BS/22 -> ToWs_Req_Bus_Sig22/1  "<testSig_DSM_bRailMeUn4Rls>"
  BS/23 -> ToWs_Req_Bus_Sig23/1  "<testSig_DSM_bRailMeUn4Blk>"
  BS/24 -> ToWs_Req_Bus_Sig24/1  "<testSig_DSM_bRailMeUn42Rls>"
  BS/25 -> ToWs_Req_Bus_Sig25/1  "<testSig_DSM_bRailMeUn42Blk>"
  BS/26 -> ToWs_Req_Bus_Sig26/1  "<testSig_DSM_bRailMeUn7Rls>"
  BS/27 -> ToWs_Req_Bus_Sig27/1  "<testSig_DSM_bRailMeUn7Blk>"
  BS/28 -> ToWs_Req_Bus_Sig28/1  "<testSig_DSM_bRailMeUn8Rls>"
  BS/29 -> ToWs_Req_Bus_Sig29/1  "<testSig_DSM_bRailMeUn8Blk>"
  BS/30 -> ToWs_Req_Bus_Sig30/1  "<testSig_DSM_bRailMeUn10Rls>"
  BS/31 -> ToWs_Req_Bus_Sig31/1  "<testSig_DSM_bRailMeUn10Blk>"
  BS/32 -> ToWs_Req_Bus_Sig32/1  "<testSig_DFC_RailMeUn0_DSM>"
  BS/33 -> ToWs_Req_Bus_Sig33/1  "<testSig_DFC_RailMeUn2_DSM>"
  BS/34 -> ToWs_Req_Bus_Sig34/1  "<testSig_DFC_RailMeUn22_DSM>"
  BS/35 -> ToWs_Req_Bus_Sig35/1  "<testSig_DFC_RailMeUn3_DSM>"
  BS/36 -> ToWs_Req_Bus_Sig36/1  "<testSig_DFC_RailMeUn4_DSM>"
  BS/37 -> ToWs_Req_Bus_Sig37/1  "<testSig_DFC_RailMeUn42_DSM>"
  BS/38 -> ToWs_Req_Bus_Sig38/1  "<testSig_DFC_RailMeUn7_DSM>"
  BS/39 -> ToWs_Req_Bus_Sig39/1  "<testSig_DFC_RailMeUn8_DSM>"
  BS/40 -> ToWs_Req_Bus_Sig40/1  "<testSig_DFC_RailMeUn10_DSM>"
  sig_Result_Bus/1 -> BS_Result/1, specifyOutputs/2(sig_Result_Bus)
  BS_Result/1 -> ToWs_Result_Bus_Sig1/1  "<DFC_RailMeUn0_DSM>"
  BS_Result/2 -> ToWs_Result_Bus_Sig2/1  "<DFC_RailMeUn2_DSM>"
  BS_Result/3 -> ToWs_Result_Bus_Sig3/1  "<DFC_RailMeUn22_DSM>"
  BS_Result/4 -> ToWs_Result_Bus_Sig4/1  "<DFC_RailMeUn3_DSM>"
  BS_Result/5 -> ToWs_Result_Bus_Sig5/1  "<DFC_RailMeUn4_DSM>"
  BS_Result/6 -> ToWs_Result_Bus_Sig6/1  "<DFC_RailMeUn42_DSM>"
  BS_Result/7 -> ToWs_Result_Bus_Sig7/1  "<DFC_RailMeUn7_DSM>"
  BS_Result/8 -> ToWs_Result_Bus_Sig8/1  "<DFC_RailMeUn8_DSM>"
  BS_Result/9 -> ToWs_Result_Bus_Sig9/1  "<DFC_RailMeUn10_DSM>"
  specifyOutputs/1(result) -> result/1

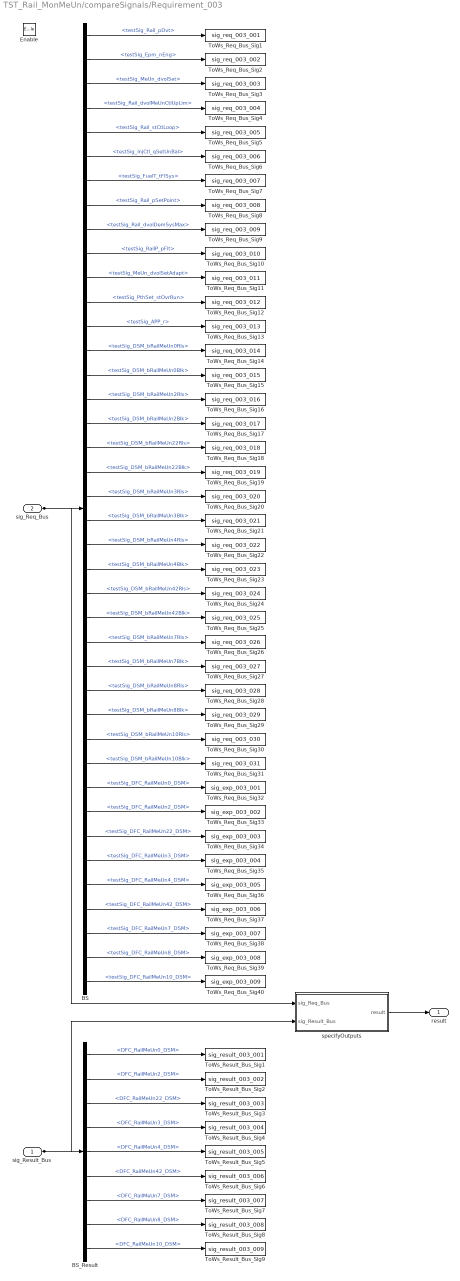
== system TST_Rail_MonMeUn/compareSignals/Requirement_003 ==
  sig_Result_Bus : Inport
  sig_Req_Bus : Inport  Port=2
  Enable : EnablePort
  BS : BusSelector  OutputSignals=testSig_Rail_pDvt,testSig_Epm_nEng,testSig_MeUn_dvolSet,testSig_Rail_dvolMeUnCtlUpLim,testSig_Rail_stCtlLoop,testSig_InjCtl_qSetUnBal,testSig_FuelT_tFlSys,testSig_Rail_pSetPoint,testSig_Rail_dvolDemSysMax,testSig_RailP_pFlt,testSig_MeUn_dvolSetAdapt,testSig_PthSet_stOvrRun,testSig_APP_r,testSig_DSM_bRailMeUn0Rls,testSig_DSM_bRailMeUn0Blk,testSig_DSM_bRailMeUn2Rls,testSig_DSM_bRailMeUn2Blk,testSig_DSM_bRailMeUn22Rls,testSig_DSM_bRailMeUn22Blk,testSig_DSM_bRailMeUn3Rls,testSig_DSM_bRailMeUn3Blk,testSig_DSM_bRailMeUn4Rls,testSig_DSM_bRailMeUn4Blk,testSig_DSM_bRailMeUn42Rls,testSig_DSM_bRailMeUn42Blk,testSig_DSM_bRailMeUn7Rls,testSig_DSM_bRailMeUn7Blk,testSig_DSM_bRailMeUn8Rls,testSig_DSM_bRailMeUn8Blk,testSig_DSM_bRailMeUn10Rls,testSig_DSM_bRailMeUn10Blk,testSig_DFC_RailMeUn0_DSM,testSig_DFC_RailMeUn2_DSM,testSig_DFC_RailMeUn22_DSM,testSig_DFC_RailMeUn3_DSM,testSig_DFC_RailMeUn4_DSM,testSig_DFC_RailMeUn42_DSM,testSig_DFC_RailMeUn7_DSM,testSig_DFC_RailMeUn8_DSM,testSig_DFC_RailMeUn10_DSM
  BS_Result : BusSelector  OutputSignals=DFC_RailMeUn0_DSM,DFC_RailMeUn2_DSM,DFC_RailMeUn22_DSM,DFC_RailMeUn3_DSM,DFC_RailMeUn4_DSM,DFC_RailMeUn42_DSM,DFC_RailMeUn7_DSM,DFC_RailMeUn8_DSM,DFC_RailMeUn10_DSM
  ToWs_Req_Bus_Sig1 : ToWorkspace  VariableName=sig_req_003_001  SaveFormat=Structure With Time
  ToWs_Req_Bus_Sig10 : ToWorkspace  VariableName=sig_req_003_010  SaveFormat=Structure With Time
  ToWs_Req_Bus_Sig11 : ToWorkspace  VariableName=sig_req_003_011  SaveFormat=Structure With Time
  ToWs_Req_Bus_Sig12 : ToWorkspace  VariableName=sig_req_003_012  SaveFormat=Structure With Time
  ToWs_Req_Bus_Sig13 : ToWorkspace  VariableName=sig_req_003_013  SaveFormat=Structure With Time
  ToWs_Req_Bus_Sig14 : ToWorkspace  VariableName=sig_req_003_014  SaveFormat=Structure With Time
  ToWs_Req_Bus_Sig15 : ToWorkspace  VariableName=sig_req_003_015  SaveFormat=Structure With Time
  ToWs_Req_Bus_Sig16 : ToWorkspace  VariableName=sig_req_003_016  SaveFormat=Structure With Time
  ToWs_Req_Bus_Sig17 : ToWorkspace  VariableName=sig_req_003_017  SaveFormat=Structure With Time
  ToWs_Req_Bus_Sig18 : ToWorkspace  VariableName=sig_req_003_018  SaveFormat=Structure With Time
  ToWs_Req_Bus_Sig19 : ToWorkspace  VariableName=sig_req_003_019  SaveFormat=Structure With Time
  ToWs_Req_Bus_Sig2 : ToWorkspace  VariableName=sig_req_003_002  SaveFormat=Structure With Time
  ToWs_Req_Bus_Sig20 : ToWorkspace  VariableName=sig_req_003_020  SaveFormat=Structure With Time
  ToWs_Req_Bus_Sig21 : ToWorkspace  VariableName=sig_req_003_021  SaveFormat=Structure With Time
  ToWs_Req_Bus_Sig22 : ToWorkspace  VariableName=sig_req_003_022  SaveFormat=Structure With Time
  ToWs_Req_Bus_Sig23 : ToWorkspace  VariableName=sig_req_003_023  SaveFormat=Structure With Time
  ToWs_Req_Bus_Sig24 : ToWorkspace  VariableName=sig_req_003_024  SaveFormat=Structure With Time
  ToWs_Req_Bus_Sig25 : ToWorkspace  VariableName=sig_req_003_025  SaveFormat=Structure With Time
  ToWs_Req_Bus_Sig26 : ToWorkspace  VariableName=sig_req_003_026  SaveFormat=Structure With Time
  ToWs_Req_Bus_Sig27 : ToWorkspace  VariableName=sig_req_003_027  SaveFormat=Structure With Time
  ToWs_Req_Bus_Sig28 : ToWorkspace  VariableName=sig_req_003_028  SaveFormat=Structure With Time
  ToWs_Req_Bus_Sig29 : ToWorkspace  VariableName=sig_req_003_029  SaveFormat=Structure With Time
  ToWs_Req_Bus_Sig3 : ToWorkspace  VariableName=sig_req_003_003  SaveFormat=Structure With Time
  ToWs_Req_Bus_Sig30 : ToWorkspace  VariableName=sig_req_003_030  SaveFormat=Structure With Time
  ToWs_Req_Bus_Sig31 : ToWorkspace  VariableName=sig_req_003_031  SaveFormat=Structure With Time
  ToWs_Req_Bus_Sig32 : ToWorkspace  VariableName=sig_exp_003_001  SaveFormat=Structure With Time
  ToWs_Req_Bus_Sig33 : ToWorkspace  VariableName=sig_exp_003_002  SaveFormat=Structure With Time
  ToWs_Req_Bus_Sig34 : ToWorkspace  VariableName=sig_exp_003_003  SaveFormat=Structure With Time
  ToWs_Req_Bus_Sig35 : ToWorkspace  VariableName=sig_exp_003_004  SaveFormat=Structure With Time
  ToWs_Req_Bus_Sig36 : ToWorkspace  VariableName=sig_exp_003_005  SaveFormat=Structure With Time
  ToWs_Req_Bus_Sig37 : ToWorkspace  VariableName=sig_exp_003_006  SaveFormat=Structure With Time
  ToWs_Req_Bus_Sig38 : ToWorkspace  VariableName=sig_exp_003_007  SaveFormat=Structure With Time
  ToWs_Req_Bus_Sig39 : ToWorkspace  VariableName=sig_exp_003_008  SaveFormat=Structure With Time
  ToWs_Req_Bus_Sig4 : ToWorkspace  VariableName=sig_req_003_004  SaveFormat=Structure With Time
  ToWs_Req_Bus_Sig40 : ToWorkspace  VariableName=sig_exp_003_009  SaveFormat=Structure With Time
  ToWs_Req_Bus_Sig5 : ToWorkspace  VariableName=sig_req_003_005  SaveFormat=Structure With Time
  ToWs_Req_Bus_Sig6 : ToWorkspace  VariableName=sig_req_003_006  SaveFormat=Structure With Time
  ToWs_Req_Bus_Sig7 : ToWorkspace  VariableName=sig_req_003_007  SaveFormat=Structure With Time
  ToWs_Req_Bus_Sig8 : ToWorkspace  VariableName=sig_req_003_008  SaveFormat=Structure With Time
  ToWs_Req_Bus_Sig9 : ToWorkspace  VariableName=sig_req_003_009  SaveFormat=Structure With Time
  ToWs_Result_Bus_Sig1 : ToWorkspace  VariableName=sig_result_003_001  SaveFormat=Structure With Time
  ToWs_Result_Bus_Sig2 : ToWorkspace  VariableName=sig_result_003_002  SaveFormat=Structure With Time
  ToWs_Result_Bus_Sig3 : ToWorkspace  VariableName=sig_result_003_003  SaveFormat=Structure With Time
  ToWs_Result_Bus_Sig4 : ToWorkspace  VariableName=sig_result_003_004  SaveFormat=Structure With Time
  ToWs_Result_Bus_Sig5 : ToWorkspace  VariableName=sig_result_003_005  SaveFormat=Structure With Time
  ToWs_Result_Bus_Sig6 : ToWorkspace  VariableName=sig_result_003_006  SaveFormat=Structure With Time
  ToWs_Result_Bus_Sig7 : ToWorkspace  VariableName=sig_result_003_007  SaveFormat=Structure With Time
  ToWs_Result_Bus_Sig8 : ToWorkspace  VariableName=sig_result_003_008  SaveFormat=Structure With Time
  ToWs_Result_Bus_Sig9 : ToWorkspace  VariableName=sig_result_003_009  SaveFormat=Structure With Time
  specifyOutputs : Subsystem
  result : Outport
  wires:
  sig_Req_Bus/1 -> BS/1, specifyOutputs/1(sig_Req_Bus)
  BS/1 -> ToWs_Req_Bus_Sig1/1  "<testSig_Rail_pDvt>"
  BS/2 -> ToWs_Req_Bus_Sig2/1  "<testSig_Epm_nEng>"
  BS/3 -> ToWs_Req_Bus_Sig3/1  "<testSig_MeUn_dvolSet>"
  BS/4 -> ToWs_Req_Bus_Sig4/1  "<testSig_Rail_dvolMeUnCtlUpLim>"
  BS/5 -> ToWs_Req_Bus_Sig5/1  "<testSig_Rail_stCtlLoop>"
  BS/6 -> ToWs_Req_Bus_Sig6/1  "<testSig_InjCtl_qSetUnBal>"
  BS/7 -> ToWs_Req_Bus_Sig7/1  "<testSig_FuelT_tFlSys>"
  BS/8 -> ToWs_Req_Bus_Sig8/1  "<testSig_Rail_pSetPoint>"
  BS/9 -> ToWs_Req_Bus_Sig9/1  "<testSig_Rail_dvolDemSysMax>"
  BS/10 -> ToWs_Req_Bus_Sig10/1  "<testSig_RailP_pFlt>"
  BS/11 -> ToWs_Req_Bus_Sig11/1  "<testSig_MeUn_dvolSetAdapt>"
  BS/12 -> ToWs_Req_Bus_Sig12/1  "<testSig_PthSet_stOvrRun>"
  BS/13 -> ToWs_Req_Bus_Sig13/1  "<testSig_APP_r>"
  BS/14 -> ToWs_Req_Bus_Sig14/1  "<testSig_DSM_bRailMeUn0Rls>"
  BS/15 -> ToWs_Req_Bus_Sig15/1  "<testSig_DSM_bRailMeUn0Blk>"
  BS/16 -> ToWs_Req_Bus_Sig16/1  "<testSig_DSM_bRailMeUn2Rls>"
  BS/17 -> ToWs_Req_Bus_Sig17/1  "<testSig_DSM_bRailMeUn2Blk>"
  BS/18 -> ToWs_Req_Bus_Sig18/1  "<testSig_DSM_bRailMeUn22Rls>"
  BS/19 -> ToWs_Req_Bus_Sig19/1  "<testSig_DSM_bRailMeUn22Blk>"
  BS/20 -> ToWs_Req_Bus_Sig20/1  "<testSig_DSM_bRailMeUn3Rls>"
  BS/21 -> ToWs_Req_Bus_Sig21/1  "<testSig_DSM_bRailMeUn3Blk>"
  BS/22 -> ToWs_Req_Bus_Sig22/1  "<testSig_DSM_bRailMeUn4Rls>"
  BS/23 -> ToWs_Req_Bus_Sig23/1  "<testSig_DSM_bRailMeUn4Blk>"
  BS/24 -> ToWs_Req_Bus_Sig24/1  "<testSig_DSM_bRailMeUn42Rls>"
  BS/25 -> ToWs_Req_Bus_Sig25/1  "<testSig_DSM_bRailMeUn42Blk>"
  BS/26 -> ToWs_Req_Bus_Sig26/1  "<testSig_DSM_bRailMeUn7Rls>"
  BS/27 -> ToWs_Req_Bus_Sig27/1  "<testSig_DSM_bRailMeUn7Blk>"
  BS/28 -> ToWs_Req_Bus_Sig28/1  "<testSig_DSM_bRailMeUn8Rls>"
  BS/29 -> ToWs_Req_Bus_Sig29/1  "<testSig_DSM_bRailMeUn8Blk>"
  BS/30 -> ToWs_Req_Bus_Sig30/1  "<testSig_DSM_bRailMeUn10Rls>"
  BS/31 -> ToWs_Req_Bus_Sig31/1  "<testSig_DSM_bRailMeUn10Blk>"
  BS/32 -> ToWs_Req_Bus_Sig32/1  "<testSig_DFC_RailMeUn0_DSM>"
  BS/33 -> ToWs_Req_Bus_Sig33/1  "<testSig_DFC_RailMeUn2_DSM>"
  BS/34 -> ToWs_Req_Bus_Sig34/1  "<testSig_DFC_RailMeUn22_DSM>"
  BS/35 -> ToWs_Req_Bus_Sig35/1  "<testSig_DFC_RailMeUn3_DSM>"
  BS/36 -> ToWs_Req_Bus_Sig36/1  "<testSig_DFC_RailMeUn4_DSM>"
  BS/37 -> ToWs_Req_Bus_Sig37/1  "<testSig_DFC_RailMeUn42_DSM>"
  BS/38 -> ToWs_Req_Bus_Sig38/1  "<testSig_DFC_RailMeUn7_DSM>"
  BS/39 -> ToWs_Req_Bus_Sig39/1  "<testSig_DFC_RailMeUn8_DSM>"
  BS/40 -> ToWs_Req_Bus_Sig40/1  "<testSig_DFC_RailMeUn10_DSM>"
  sig_Result_Bus/1 -> BS_Result/1, specifyOutputs/2(sig_Result_Bus)
  BS_Result/1 -> ToWs_Result_Bus_Sig1/1  "<DFC_RailMeUn0_DSM>"
  BS_Result/2 -> ToWs_Result_Bus_Sig2/1  "<DFC_RailMeUn2_DSM>"
  BS_Result/3 -> ToWs_Result_Bus_Sig3/1  "<DFC_RailMeUn22_DSM>"
  BS_Result/4 -> ToWs_Result_Bus_Sig4/1  "<DFC_RailMeUn3_DSM>"
  BS_Result/5 -> ToWs_Result_Bus_Sig5/1  "<DFC_RailMeUn4_DSM>"
  BS_Result/6 -> ToWs_Result_Bus_Sig6/1  "<DFC_RailMeUn42_DSM>"
  BS_Result/7 -> ToWs_Result_Bus_Sig7/1  "<DFC_RailMeUn7_DSM>"
  BS_Result/8 -> ToWs_Result_Bus_Sig8/1  "<DFC_RailMeUn8_DSM>"
  BS_Result/9 -> ToWs_Result_Bus_Sig9/1  "<DFC_RailMeUn10_DSM>"
  specifyOutputs/1(result) -> result/1
